simulink model "Copy_of_untitled"  (R2015a)
settings: Solver=ode45  StartTime=0.0  StopTime=1800  RelTol=1e-3
libraries: simulink x1
settings Model: Creator=christian  LastModifiedBy=christian

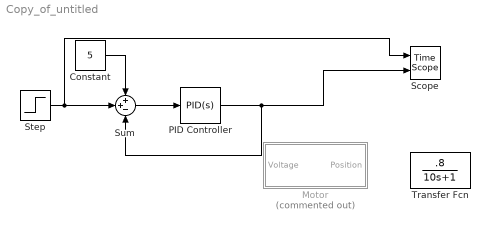
== system Copy_of_untitled ==
  Constant : Constant  Value=5
  Motor : Subsystem  Commented=on
  PID Controller : simulink/Continuous/PID Controller  Controller=PID  TimeDomain=Continuous-time  SampleTime=-1  IntegratorMethod=Forward Euler  FilterMethod=Forward Euler  Form=Parallel  UseFilter=on  ControllerParametersSource=internal  P=0  I=1e-3  D=0  N=1  InitialConditionSource=internal  InitialConditionForIntegrator=0  InitialConditionForFilter=0  ExternalReset=none  LimitOutput=off  UpperSaturationLimit=40.3  LowerSaturationLimit=40  LinearizeAsGain=on  AntiWindupMode=none  Kb=1  TrackingMode=off  Kt=1  PParamMin=[]  PParamMax=[]  IParamMin=[]  IParamMax=[]  DParamMin=[]  DParamMax=[]  NParamMin=[]  NParamMax=[]  KbParamMin=[]  KbParamMax=[]  KtParamMin=[]  KtParamMax=[]  POutMin=[]  POutMax=[]  IOutMin=[]  IOutMax=[]  DOutMin=[]  DOutMax=[]  NOutMin=[]  NOutMax=[]  KbOutMin=[]  KbOutMax=[]  KtOutMin=[]  KtOutMax=[]  IntegratorOutMin=[]  IntegratorOutMax=[]  FilterOutMin=[]  FilterOutMax=[]  SumOutMin=[]  SumOutMax=[]  SumI1OutMin=[]  SumI1OutMax=[]  SumI2OutMin=[]  SumI2OutMax=[]  SumI3OutMin=[]  SumI3OutMax=[]  SumDOutMin=[]  SumDOutMax=[]  SaturationOutMin=[]  SaturationOutMax=[]  IntegratorContinuousStateAttributes=''  IntegratorStateMustResolveToSignalObject=off  IntegratorRTWStateStorageClass=Auto  FilterContinuousStateAttributes=''  FilterStateMustResolveToSignalObject=off  FilterRTWStateStorageClass=Auto  DifferentiatorICPrevScaledInput=0  DifferentiatorOutMin=[]  DifferentiatorOutMax=[]
  Scope : TimeScope  NumInputPorts=2
  Step : Step  Time=300  After=.5  SampleTime=0
  Sum : Sum  Inputs=++-
  Transfer Fcn : TransferFcn  Numerator=[.8]  Denominator=[10 1]
  wires:
  Sum/1 -> PID Controller/1
  Step/1 -> Sum/2, Scope/1
  PID Controller/1 -> Scope/2, Sum/3
  Constant/1 -> Sum/1

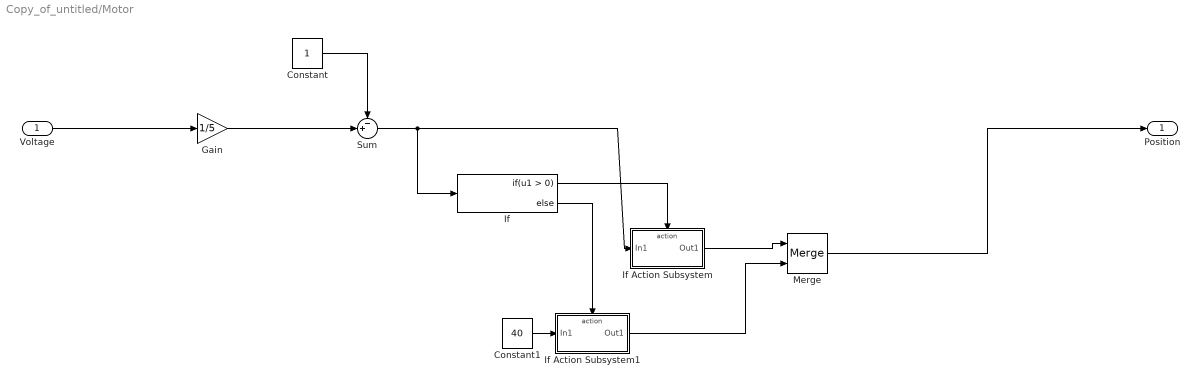
== system Copy_of_untitled/Motor ==
  Voltage : Inport
  Constant : Constant
  Constant1 : Constant  Value=40
  Gain : Gain  Gain=1/5
  If : If
  If Action Subsystem : Subsystem  TreatAsAtomicUnit=on
  If Action Subsystem1 : Subsystem  TreatAsAtomicUnit=on
  Merge : Merge
  Sum : Sum  Inputs=-+|
  Position : Outport
  wires:
  Voltage/1 -> Gain/1
  Gain/1 -> Sum/2
  Constant/1 -> Sum/1
  Merge/1 -> Position/1
  If/1 -> If Action Subsystem/Action
  If Action Subsystem/1(Out1) -> Merge/1
  If/2 -> If Action Subsystem1/Action
  If Action Subsystem1/1(Out1) -> Merge/2
  Constant1/1 -> If Action Subsystem1/1(In1)
  Sum/1 -> If/1, If Action Subsystem/1(In1)

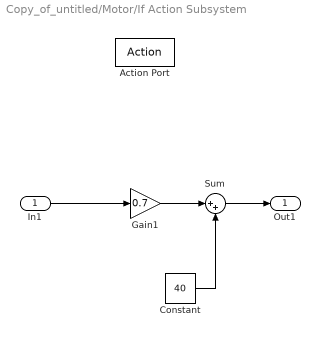
== system Copy_of_untitled/Motor/If Action Subsystem ==
  In1 : Inport
  Action Port : ActionPort
  Constant : Constant  Value=40
  Gain1 : Gain  Gain=0.7
  Sum : Sum  Inputs=|++
  Out1 : Outport
  wires:
  In1/1 -> Gain1/1
  Gain1/1 -> Sum/1
  Sum/1 -> Out1/1
  Constant/1 -> Sum/2

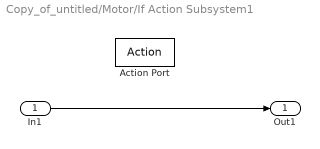
== system Copy_of_untitled/Motor/If Action Subsystem1 ==
  In1 : Inport
  Action Port : ActionPort
  Out1 : Outport
  wires:
  In1/1 -> Out1/1
